simulink model "boost_conv"  (R2024b)
settings: Solver=VariableStepAuto  StartTime=0.0  StopTime=100.0  RelTol=1e-3
libraries: cstblocks x4
settings Model: Creator=kuv2707  LastModifiedBy=kuv2707

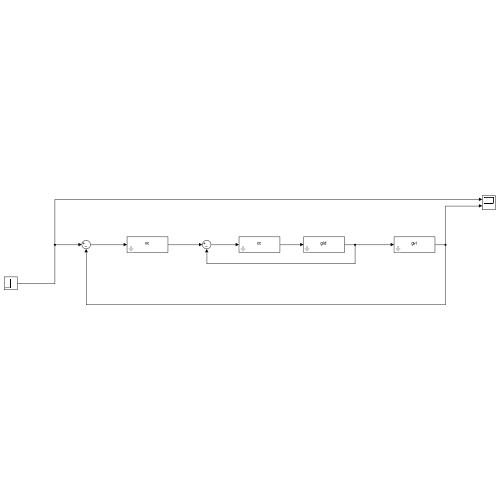
[thumbnail: Simulink's stored preview of the top-level diagram]
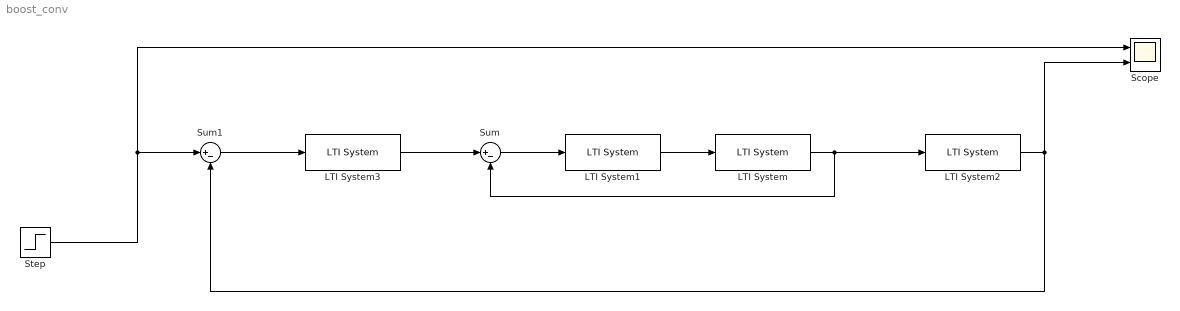
== system boost_conv ==
  LTI System : cstblocks/LTI System  sys=gid  IC=[]  PadeOrder=0
  LTI System1 : cstblocks/LTI System  sys=cc  IC=[]  PadeOrder=0
  LTI System2 : cstblocks/LTI System  sys=gvi  IC=[]  PadeOrder=0
  LTI System3 : cstblocks/LTI System  sys=vc  IC=[]  PadeOrder=0
  Scope : Scope  NumInputPorts=2
  Step : Step  After=10  SampleTime=0
  Sum : Sum  Inputs=|+-
  Sum1 : Sum  Inputs=|+-
  wires:
  LTI System1/1 -> LTI System/1
  Sum/1 -> LTI System1/1
  LTI System/1 -> LTI System2/1, Sum/2
  LTI System3/1 -> Sum/1
  Sum1/1 -> LTI System3/1
  LTI System2/1 -> Scope/2, Sum1/2
  Step/1 -> Scope/1, Sum1/1
